simulink model "sldemo_tc"  (R2024a)
settings: Solver=ode3  StartTime=0.0  StopTime=10.0  FixedStep=0.005  RelTol=1e-3
StartFcn:
  | set_param('sldemo_tc/Scope','Open','on')
model workspace (MAT data in the model file):
  TypeS_E_Volts = [-0.000236 -0.000232 -0.000228 -0.000224 -0.000219 -0.000215 -0.000211 -0.000207 -0.000203 -0.000199 -0.000194 -0.00019 ... (1816 elements, 1816x1)]
  TypeS_T_degC = [-50 -49 -48 -47 -46 -45 -44 -43 -42 -41 -40 -39 ... (1816 elements, 1816x1)]
  TypeS_bits_bp = [0; 50; 100; 150; 200; 250; 300; 350; 400; 450; 500; 550; 600; 650; 700; 750; 800; 850; 900; 950; 1000; 1050; 1100; 1150; 1200; 1250; 1300; 1350; 1400; 1450; 1500; 1550; 1600; 1650; 1700; 1750; 1800; 1850; 1900; 1950; 2000; 2050; 2100; 2150; 2200; 2250; 2300; 2350; 2400; 2450; 2500; 2550; 2600; 2650; 2700; 2750; 2800; 2850; 2900; 2950; 3000; 3050; 3100; 3150; 3200; 3250; 3300; 3350; 3400; 3450; 3500; 3550; 3600; 3650; 3700; 3750; 3800; 3850; 3900; 3950; 4000; 4050; 4095]
  TypeS_tdegc_interp = [-50; -1.05395507812; 38.4789352417; 73.4326858521; 105.529296875; 135.797668457; 164.757202148; 192.63710022; 219.712234497; 246.231826782; 272.095336914; 297.6043396; 322.790588379; 347.53237915; 372.051971436; 396.31439209; 420.382019043; 444.149658203; 467.81729126; 491.284912109; 514.55255127; 537.620178223; 560.587768555; 583.355407715; 606.023071289; 628.490661621; 650.858276367; 673.02355957; 694.994140625; 716.873779297; 738.62878418; 760.178588867; 781.60369873; 802.846984863; 823.999389648; 844.969970703; 865.849609375; 886.547424316; 907.15435791; 927.614562988; 948.004211426; 968.227233887; 988.309387207; 1008.27996826; 1028.22961426; 1047.95263672; 1067.67565918; 1087.23205566; 1106.76916504; 1126.17810059; 1145.56774902; 1164.79077148; 1184.09716797; 1203.23681641; 1222.37658691; 1241.51623535; 1260.57263184; 1279.62890625; 1298.68530273; 1317.74169922; 1336.71472168; 1355.71166992; 1374.74401855; 1393.71704102; 1412.7734375; 1431.82983398; 1450.8861084; 1469.94250488; 1489.08215332; 1508.22192383; 1527.44494629; 1546.66796875; 1565.97424316; 1585.36401367; 1604.83703613; 1624.33825684; 1643.94970703; 1663.67272949; 1683.47912598; 1703.49316406; 1723.91833496; 1744.9777832; 1764.53869629]
  TypeS_tdegc_vs_bits = [-50 -48.8466186523 -47.6932373047 -46.6318855286 -45.6364746094 -44.4830932617 -43.3297119141 -42.1763305664 -41.0229492188 -40.0956535339 -38.9661865234 -37.8502426147 ... (4096 elements, 4096x1)]
  e_vs_counts = [-0.236 -0.231386474609 -0.226772949219 -0.222159423828 -0.217545898437 -0.212932373047 -0.208318847656 -0.203705322266 -0.199091796875 -0.194478271484 -0.189864746094 -0.185251220703 ... (4096 elements, 4096x1)]
libraries: simulink_extras x1
(part 1 of 2)
Description:
  | Thermocouple Modeling and Signal Conversion
  | 
  | The thermocouple is one of the popular analog transducers today, along
  | with other devices such as position sensors, strain gages, pressure
  | transducers, and resistance temperature devices (RTDs). Operating under
  | the principle of the Seebeck (or thermoelectric) effect, thermocouples
  | have an empirically determined nonlinear behavior that is well known over
  | each junction type's useful operating range. If you run the model, you
  | will be able to see the cumulative effect of each component on dynamic
  | measurement accuracy. This demonstration will focus on models for each of
  | these components in a dynamic temperature measurement system for a Type S
  | (Platinum-10% Rhodium(+) versus Platinum(-) ) : a thermocouple device and
  | probe assembly, a signal conditioning method, an analog to digital
  | converter (ADC), and a software specification for converting the ADC
  | output back into a temperature value. An additional section shows how to
  | obtain and use standard NIST ITS-90 thermocouple data with Simulink
  | models. Look-up tables and a polynomial block are used in this design to
  | capture the nonlinear behavior of the thermocouple. Note that the
  | polynomial block is a viable alternative to look-up tables for some
  | applications, minimizing ROM usage at the cost of some additional
  | computation for the full polynomial representation.
settings Model: Creator=The MathWorks, Inc.  LastModifiedBy=neham
settings SolverCC: AlgebraicLoopSolver=TrustRegion
settings DataIOCC: LimitDataPoints=on  SaveFormat=Array  SaveOutput=off  SaveTime=off
settings OptimizationCC: DefaultParameterBehavior=Inlined  InlineInvariantSignals=on  ExpressionDepthLimit=2147483647  InitFltsAndDblsToZero=on  LifeSpan=inf  BufferReusableBoundary=off
settings DebuggingCC: SaveWithParameterizedLinksMsg=none  UnderspecifiedInitializationDetection=Classic  MergeDetectMultiDrivingBlocksExec=none  CheckExecutionContextPreStartOutputMsg=on  SignalResolutionControl=TryResolveAllWithWarning  SolverPrmCheckMsg=warning  MultiTaskDSMMsg=warning  MultiTaskCondExecSysMsg=none  FcnCallInpInsideContextMsg=warning  UnconnectedInputMsg=warning  UnconnectedOutputMsg=warning  UnconnectedLineMsg=warning  BusObjectLabelMismatch=none  StateNameClashWarn=warning  SFUnexpectedBacktrackingDiag=warning  SFNoUnconditionalDefaultTransitionDiag=warning  SFExecutionAtInitializationDiag=none  ArithmeticOperatorsInVariantConditions=warning
settings HardwareCC: ProdBitPerPointer=32  ProdBitPerSizeT=32  ProdBitPerPtrDiffT=32  ProdLargestAtomicFloat=None  ProdIntDivRoundTo=Floor  ProdWordSize=32  ProdHWDeviceType=32-bit xPC Target (AMD Athlon)
settings ModelReferenceCC: EnableRefExpFcnMdlSchedulingChecks=on  PropagateSignalLabelsOutOfModel=off
settings SFSimCC: SimUseLocalCustomCode=off  CustomCodeUndefinedFunction=UseInterfaceOnly
settings RTWCC: GenCodeOnly=on  RTWUseLocalCustomCode=off  GPUComputeCapability=3.5
settings CodeAppCC: StateflowObjectComments=on
settings GRTTargetCC: TargetFcnLib=iso_tfl_tmw.mat  CombineOutputUpdateFcns=off  GRTInterface=on
settings ConfigComp: CovMetricSettings=dw  CovSaveCumulativeToWorkspaceVar=on  CovSaveSingleToWorkspaceVar=on  CovExternalEMLEnable=off

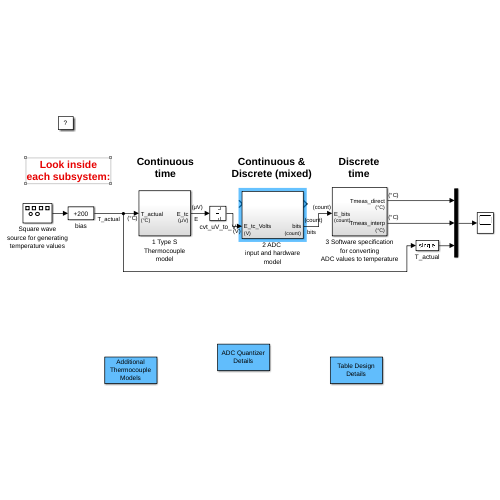
[thumbnail: Simulink's stored preview of the top-level diagram]
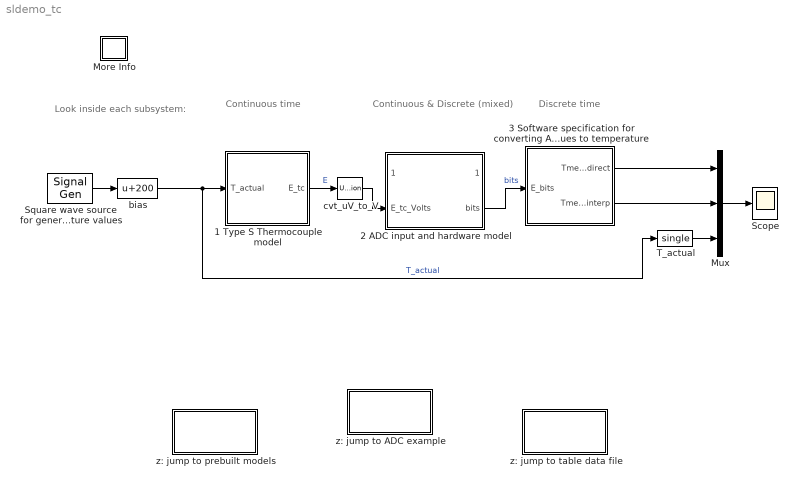
== system sldemo_tc ==
  note: Continuous
      | time
  note: Discrete
      | time
  note: Continuous &
      | Discrete (mixed)
  note: Look inside
      | each subsystem:
  1 Type S Thermocouple model : Subsystem
  2 ADC input and hardware model : Subsystem
  3 Software specification for converting ADC values to temperature : Subsystem
  More Info : Subsystem
      settings: OpenFcn=showExample('simulink_general/sldemo_tc_scriptExample')
      mask Display: disp('?')
  Mux : Mux  Inputs=3
  Scope : Scope
  Square wave source for generating temperature values : SignalGenerator  WaveForm=square  Amplitude=100
  T_actual : DataTypeConversion  OutDataTypeStr=single  SaturateOnIntegerOverflow=off  RndMeth=Floor
  bias : Bias  Bias=200  SaturateOnIntegerOverflow=off
  cvt_uV_to_V : UnitConversion
  z: jump to ADC example : Subsystem  mask(ADC quantizer details){}
      mask help: Jump to a model that exercises more details of the behavior of the Idealized ADC quantizer block that is part of the hardware model.
      settings: OpenFcn=open_system('sldemo_adc_quantize','force')
      mask Display: disp('ADC Quantizer\nDetails')
  z: jump to prebuilt models : Subsystem  mask(ADC quantizer details){}
      mask help: Jump to a model that exercises more details of the behavior of the Idealized ADC quantizer block that is part of the hardware model.
      settings: OpenFcn=open_system('sldemo_tc_blocks','force')
      mask Display: disp('Additional\nThermocouple\nModels')
  z: jump to table data file : Subsystem  mask(ADC quantizer details){}
      mask help: Jump to a model that exercises more details of the behavior of the Idealized ADC quantizer block that is part of the hardware model.
      settings: OpenFcn=edit sldemo_create_tc_tabledata.m
      mask Display: disp('Table Design\nDetails')
  wires:
  3 Software specification for converting ADC values to temperature/1(Tmeas_direct) -> Mux/1
  1 Type S Thermocouple model/1(E_tc) -> cvt_uV_to_V/1  "E"
  2 ADC input and hardware model/2(bits) -> 3 Software specification for converting ADC values to temperature/1(E_bits)  "bits"
  3 Software specification for converting ADC values to temperature/2(Tmeas_interp) -> Mux/2
  Mux/1 -> Scope/1
  bias/1 -> 1 Type S Thermocouple model/1(T_actual), T_actual/1  "T_actual"
  Square wave source for generating temperature values/1 -> bias/1
  T_actual/1 -> Mux/3
  cvt_uV_to_V/1 -> 2 ADC input and hardware model/2(E_tc_Volts)
